simulink model "Microgrid"  (R2025b)
settings: Solver=FixedStepAuto  StartTime=0.0  StopTime=1  FixedStep=5e-7  RelTol=1e-3
InitFcn:
  | unitlmModelFile = get_param(bdroot, 'FileName');
  | if ~isempty(unitlmModelFile), addpath(fileparts(unitlmModelFile)); end
  | initialize_unitlm_microgrid();
  | clear unitlmModelFile
StopFcn:
  | %% StopFcn: save reference-system simulation results
  | 
  | % 获取模型文件所在目录
  | modelName = bdroot;
  | modelFile = get_param(modelName, 'FileName');
  | 
  | if isempty(modelFile)
  |     % 模型尚未保存时，使用当前工作目录
  |     modelDir = pwd;
  | else
  |     modelDir = fileparts(modelFile);
  | end
  | 
  | % 创建 result 文件夹
  | resultDir = fullfile(modelDir, 'result');
  | 
  | if ~exist(resultDir, 'dir')
  |     mkdir(resultDir);
  | end
  | 
  | % 需要保存的工作区变量
  | variableNames = {
  |     'server_voltage'
  |     'server_current'
  |     'server_PQ'
  |     'client_voltage'
  |     'client_current'
  |     'client_PQ'
  |     'client_omega'
  | };
  | 
  | % 用结构体保存，并添加 _ref 后缀
  | refData = struct();
  | 
  | for k = 1:numel(variableNames)
  | 
  |     originalName = variableNames{k};
  |     refName      = [originalName, '_ref'];
  | 
  |     % 检查变量是否存在于 Base Workspace
  |     variableExists = evalin( ...
  |         'base', ...
  |         sprintf('exist(''%s'', ''var'')', originalName));
  | 
  |     if variableExists
  |         refData.(refName) = evalin('base', originalName);
  |     else
  |         warning( ...
  |             'StopFcn:MissingVariable', ...
  |             'Variable "%s" was not found in the base workspace.', ...
  |             originalName);
  |     end
  | end
  | 
  | % 保存为 result/ref_system.mat
  | saveFile = fullfile(resultDir, 'ref_system.mat');
  | save(saveFile, '-struct', 'refData');
  | 
  | fprintf('Reference-system results saved to:\n%s\n', saveFile);
values from neighbouring files (symbols this model uses):
  Cf = Cf_pu*Cb    [initialize_unitlm_microgrid.m]
  f = logspace(log10(fMin), log10(fMax), nFrequency).'    [fit_non_heaviside_line_rational.m]    (also in initialize_unitlm_microgrid.m = 50)
  fsw1 = 10e3    (= 10000)    [initialize_unitlm_microgrid.m]
  gfm_AngleKi = 3    [initialize_unitlm_microgrid.m]
  gfm_AngleKp = 1.2    [initialize_unitlm_microgrid.m]
  gfm_PrefPu = 1.0    (= 1)    [initialize_unitlm_microgrid.m]
  gfm_VloopKi = 120    [initialize_unitlm_microgrid.m]
  gfm_VloopKp = 0.08    [initialize_unitlm_microgrid.m]
  gfm_VrefPu = 0.93    [initialize_unitlm_microgrid.m]
  Ip = 2*P/(3*Vp)    [initialize_unitlm_microgrid.m]
  L1 = L1_pu*Lb    [initialize_unitlm_microgrid.m]
  L2 = L2_pu*Lb    [initialize_unitlm_microgrid.m]
  L3 = L3_pu*Lb    [initialize_unitlm_microgrid.m]
  L4 = L4_pu*Lb    [initialize_unitlm_microgrid.m]
  Lc = Lc_pu*Lb    [initialize_unitlm_microgrid.m]
  Lf2 = Lf2_pu*Lb    [initialize_unitlm_microgrid.m]
  P = 5e6    (= 5000000)    [initialize_unitlm_microgrid.m]
  R1 = R1_pu*Zb    [initialize_unitlm_microgrid.m]
  R2 = R2_pu*Zb    [initialize_unitlm_microgrid.m]
  R3 = R3_pu*Zb    [initialize_unitlm_microgrid.m]
  R4 = R4_pu*Zb    [initialize_unitlm_microgrid.m]
  Rdamp = Rf    [initialize_unitlm_microgrid.m]
  Rf = Rf_pu*Zb    [initialize_unitlm_microgrid.m]
  Rload1 = Vp/Ip    [initialize_unitlm_microgrid.m]
  Rload2 = Vp/Ip    [initialize_unitlm_microgrid.m]
  Rload3 = Vp/Ip    [initialize_unitlm_microgrid.m]
  Rv_pu = 0.1    [initialize_unitlm_microgrid.m]
  Sxfmr = 6.3e6    (= 6300000)    [initialize_unitlm_microgrid.m]
  Vac = sqrt(2)*Vline/sqrt(3)    [initialize_unitlm_microgrid.m]
  Vdc = 1350    [initialize_unitlm_microgrid.m]
  Vhv = 66e3    (= 66000)    [initialize_unitlm_microgrid.m]
  Vline = 690    [initialize_unitlm_microgrid.m]
  Vp = Vac    [initialize_unitlm_microgrid.m]
  Wb = 2*pi*f    (= 314.159265359)    [initialize_unitlm_microgrid.m]
  Xv_pu = 0.3    [initialize_unitlm_microgrid.m]
undefined symbols (not defined in the file or in its folder): DiscIntNeverNeededParam, DPL, Lline1
libraries: spsThreePhaseSeriesRLCBranchLib x17, spsControlledVoltageSourceLib x9, spsabctodq0Lib x9, spsThreePhaseVIMeasurementLib x8, slpidlib x7, spsPower3phInstantaneousLib x4, spsThreePhaseBreakerLib x4, spsThreePhaseTransformerTwoWindingsLib x4, spsdq0toabcLib x3, SimplusGT x3, spsDCVoltageSourceLib x1, spsDistributedParametersLineLib x1
(part 3 of 3)

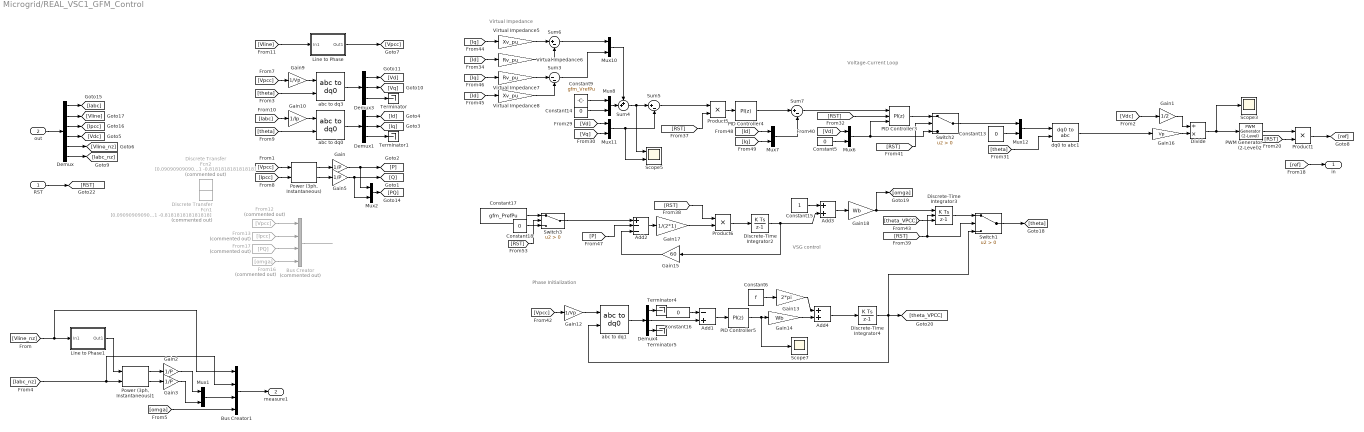
== system Microgrid/REAL_VSC1_GFM_Control ==
  note: Voltage-Current Loop
  note: VSG control
  note: Virtual Impedance
  note: Phase Initialization
  RST : Inport
  out : Inport  Port=2
  Add1 : Sum  Inputs=-+
  Add2 : Sum  Inputs=+--
  Add3 : Sum
  Add4 : Sum
  Bus Creator : BusCreator  Commented=on  Inputs=4
  Bus Creator1 : BusCreator  Inputs=4
  Constant{5,13..14,16} (4 alike) : Constant  Value=0
  Constant15 : Constant
  Constant17 : Constant  Value=gfm_PrefPu  SampleTime=-1
  Constant18 : Constant  Value=0  SampleTime=-1
  Constant6 : Constant  Value=f
  Constant9 : Constant  Value=gfm_VrefPu  SampleTime=-1
  Demux : Demux  Outputs=6
  Demux1 : Demux  Outputs=3
  Demux3 : Demux  Outputs=3
  Demux4 : Demux  Outputs=3
  Discrete Transfer Fcn1 : DiscreteTransferFcn  Commented=on  Numerator=[0.090909090909091 0.090909090909091]  Denominator=[1 -0.818181818181818]
  Discrete Transfer Fcn2 : DiscreteTransferFcn  Commented=on  Numerator=[0.090909090909091 0.090909090909091]  Denominator=[1 -0.818181818181818]
  Discrete-Time Integrator2 : DiscreteIntegrator  SampleTime=1/fsw1  ICPrevOutput=DiscIntNeverNeededParam  ICPrevScaledInput=DiscIntNeverNeededParam
  Discrete-Time Integrator3 : DiscreteIntegrator  ExternalReset=rising  InitialConditionSource=external  SampleTime=1/fsw1  ICPrevOutput=DiscIntNeverNeededParam  ICPrevScaledInput=DiscIntNeverNeededParam
  Discrete-Time Integrator4 : DiscreteIntegrator  SampleTime=1/fsw1  ICPrevOutput=DiscIntNeverNeededParam  ICPrevScaledInput=DiscIntNeverNeededParam
  Divide : Product  Inputs=/*
  From12 : From  Commented=on  GotoTag=Vpcc
  From13 : From  Commented=on  GotoTag=Ipcc
  From16 : From  Commented=on  GotoTag=omga
  From17 : From  Commented=on  GotoTag=PQ
  Gain{,2..3,5} (4 alike) : Gain  Gain=1/P
  Gain1 : Gain  Gain=1/2
  Gain10 : Gain  Gain=1/Ip
  Gain12 : Gain  Gain=1/Vp
  Gain13 : Gain  Gain=2*pi
  Gain14 : Gain  Gain=Wb
  Gain15 : Gain  Gain=60
  Gain16 : Gain  Gain=Vp
  Gain17 : Gain  Gain=1/(2*1)
  Gain18 : Gain  Gain=Wb
  Gain9 : Gain  Gain=1/Vp
  Line to Phase : Subsystem
  Line to Phase1 : Subsystem
  Mux{1..2,6..8,10..12} (8 alike) : Mux  Inputs=2
  PID Controller3 : slpidlib/PID Controller  Controller=PI  Form=Parallel  TimeDomain=Discrete-time  UseExternalTs=off  SampleTime=1/fsw1  IntegratorMethod=Forward Euler  FilterMethod=Forward Euler  ControllerParametersSource=internal  P=0.5  I=100  UseKiTs=off  D=0  UseExternalDerivativeSource=off  N=100  UseFilter=on  TunerSelectOption=Transfer Function Based (PID Tuner App)  InitialConditionSource=external  InitialConditionForIntegrator=0  InitialConditionForFilter=0  DifferentiatorICPrevScaledInput=0  ExternalReset=rising  TrackingMode=off  Kt=1  LimitOutput=off  SatLimitsSource=internal  UpperSaturationLimit=inf  LowerSaturationLimit=-inf  LinearizeAsGain=on  AntiWindupMode=none  Kb=1  LimitIntegrator=off  UpperIntegratorSaturationLimit=inf  LowerIntegratorSaturationLimit=-inf  POutMin=[]  POutMax=[]  IOutMin=[]  IOutMax=[]  DOutMin=[]  DOutMax=[]  NOutMin=[]  NOutMax=[]  SumOutMin=[]  SumOutMax=[]  SaturationOutMin=[]  SaturationOutMax=[]  PParamMin=[]  PParamMax=[]  IParamMin=[]  IParamMax=[]  DParamMin=[]  DParamMax=[]  NParamMin=[]  NParamMax=[]  KbParamMin=[]  KbParamMax=[]  KtParamMin=[]  KtParamMax=[]  KbOutMin=[]  KbOutMax=[]  KtOutMin=[]  KtOutMax=[]  IntegratorOutMin=[]  IntegratorOutMax=[]  FilterOutMin=[]  FilterOutMax=[]  SumI1OutMin=[]  SumI1OutMax=[]  SumI2OutMin=[]  SumI2OutMax=[]  SumI3OutMin=[]  SumI3OutMax=[]  SumI4OutMin=[]  SumI4OutMax=[]  SumDOutMin=[]  SumDOutMax=[]  DifferentiatorOutMin=[]  DifferentiatorOutMax=[]  FilterDiffOutCoefMin=[]  FilterDiffOutCoefMax=[]  ReciprocalOutMin=[]  ReciprocalOutMax=[]  SumDenOutMin=[]  SumDenOutMax=[]  SumNumOutMin=[]  SumNumOutMax=[]  DivideOutMin=[]  DivideOutMax=[]  UdiffTsProdOutMin=[]  UdiffTsProdOutMax=[]  NTsProdOutMin=[]  NTsProdOutMax=[]  UintegralTsProdOutMin=[]  UintegralTsProdOutMax=[]  UngainTsProdOutMin=[]  UngainTsProdOutMax=[]  ClampingZeroOutDataTypeStr=Inherit: Inherit via back propagation  ClampingZeroOutMin=[]  ClampingZeroOutMax=[]  FilterDenConstantOutDataTypeStr=Inherit: Inherit via back propagation  FilterDenConstantOutMin=[]  FilterDenConstantOutMax=[]  PCopyOutDataTypeStr=Inherit: Inherit via back propagation  PCopyOutMin=[]  PCopyOutMax=[]  NCopyOutDataTypeStr=Inherit: Inherit via back propagation  NCopyOutMin=[]  NCopyOutMax=[]  IntegratorContinuousStateAttributes=''  IntegratorStateMustResolveToSignalObject=off  IntegratorRTWStateStorageClass=Auto  FilterContinuousStateAttributes=''  FilterStateMustResolveToSignalObject=off  FilterRTWStateStorageClass=Auto  ParallelPVariant=InternalParameters  IdealPVariant=Disabled  IVariant=InternalParameters  DVariant=Disabled  IntegratorVariant=Discrete  SatVariant=Disabled  AWVariant=Passthrough  PCopyVariant=Disabled  TRVariant=Disabled  FdbkBlocksVariant=Forward  IdealPFdbkVariant=Disabled  SatFdbkVariant=Disabled  DerivativeFilterVariant=Disabled  NVariant=Disabled  NCopyVariant=Disabled_SignalSpec  FilterICVariant=Disabled  IntegratorICVariant=ExternalICs  ExternalResetVariant=ExternalReset  TRSumVariant=Passthrough  SumFdbkVariant=Disabled  SumVariant=Sum_PI  TsampFilterVariant=InternalTs  TsampNgainVariant=Passthrough  TsampIntegralVariant=Disabled_SignalSpec  ExternalSaturationOutDataTypeStr=Inherit: Same as second input  DerivativeSourceVariant=Disabled  PreIntVariant=InternalPreInt
  PID Controller4 : slpidlib/PID Controller  Controller=PI  Form=Parallel  TimeDomain=Discrete-time  UseExternalTs=off  SampleTime=1/fsw1  IntegratorMethod=Forward Euler  FilterMethod=Forward Euler  ControllerParametersSource=internal  P=gfm_VloopKp  I=gfm_VloopKi  UseKiTs=off  D=0  UseExternalDerivativeSource=off  N=100  UseFilter=on  TunerSelectOption=Transfer Function Based (PID Tuner App)  InitialConditionSource=internal  InitialConditionForIntegrator=0  InitialConditionForFilter=0  DifferentiatorICPrevScaledInput=0  ExternalReset=none  TrackingMode=off  Kt=1  LimitOutput=off  SatLimitsSource=internal  UpperSaturationLimit=inf  LowerSaturationLimit=-inf  LinearizeAsGain=on  AntiWindupMode=none  Kb=1  LimitIntegrator=off  UpperIntegratorSaturationLimit=inf  LowerIntegratorSaturationLimit=-inf  POutMin=[]  POutMax=[]  IOutMin=[]  IOutMax=[]  DOutMin=[]  DOutMax=[]  NOutMin=[]  NOutMax=[]  SumOutMin=[]  SumOutMax=[]  SaturationOutMin=[]  SaturationOutMax=[]  PParamMin=[]  PParamMax=[]  IParamMin=[]  IParamMax=[]  DParamMin=[]  DParamMax=[]  NParamMin=[]  NParamMax=[]  KbParamMin=[]  KbParamMax=[]  KtParamMin=[]  KtParamMax=[]  KbOutMin=[]  KbOutMax=[]  KtOutMin=[]  KtOutMax=[]  IntegratorOutMin=[]  IntegratorOutMax=[]  FilterOutMin=[]  FilterOutMax=[]  SumI1OutMin=[]  SumI1OutMax=[]  SumI2OutMin=[]  SumI2OutMax=[]  SumI3OutMin=[]  SumI3OutMax=[]  SumI4OutMin=[]  SumI4OutMax=[]  SumDOutMin=[]  SumDOutMax=[]  DifferentiatorOutMin=[]  DifferentiatorOutMax=[]  FilterDiffOutCoefMin=[]  FilterDiffOutCoefMax=[]  ReciprocalOutMin=[]  ReciprocalOutMax=[]  SumDenOutMin=[]  SumDenOutMax=[]  SumNumOutMin=[]  SumNumOutMax=[]  DivideOutMin=[]  DivideOutMax=[]  UdiffTsProdOutMin=[]  UdiffTsProdOutMax=[]  NTsProdOutMin=[]  NTsProdOutMax=[]  UintegralTsProdOutMin=[]  UintegralTsProdOutMax=[]  UngainTsProdOutMin=[]  UngainTsProdOutMax=[]  ClampingZeroOutDataTypeStr=Inherit: Inherit via back propagation  ClampingZeroOutMin=[]  ClampingZeroOutMax=[]  FilterDenConstantOutDataTypeStr=Inherit: Inherit via back propagation  FilterDenConstantOutMin=[]  FilterDenConstantOutMax=[]  PCopyOutDataTypeStr=Inherit: Inherit via back propagation  PCopyOutMin=[]  PCopyOutMax=[]  NCopyOutDataTypeStr=Inherit: Inherit via back propagation  NCopyOutMin=[]  NCopyOutMax=[]  IntegratorContinuousStateAttributes=''  IntegratorStateMustResolveToSignalObject=off  IntegratorRTWStateStorageClass=Auto  FilterContinuousStateAttributes=''  FilterStateMustResolveToSignalObject=off  FilterRTWStateStorageClass=Auto  ParallelPVariant=InternalParameters  IdealPVariant=Disabled  IVariant=InternalParameters  DVariant=Disabled  IntegratorVariant=Discrete  SatVariant=Disabled  AWVariant=Passthrough  PCopyVariant=Disabled  TRVariant=Disabled  FdbkBlocksVariant=Forward  IdealPFdbkVariant=Disabled  SatFdbkVariant=Disabled  DerivativeFilterVariant=Disabled  NVariant=Disabled  NCopyVariant=Disabled_SignalSpec  FilterICVariant=Disabled  IntegratorICVariant=InternalICs  ExternalResetVariant=Disabled  TRSumVariant=Passthrough  SumFdbkVariant=Disabled  SumVariant=Sum_PI  TsampFilterVariant=InternalTs  TsampNgainVariant=Passthrough  TsampIntegralVariant=Disabled_SignalSpec  ExternalSaturationOutDataTypeStr=Inherit: Same as second input  DerivativeSourceVariant=Disabled  PreIntVariant=InternalPreInt
  PID Controller5 : slpidlib/PID Controller  Controller=PI  Form=Parallel  TimeDomain=Discrete-time  UseExternalTs=off  SampleTime=1/fsw1  IntegratorMethod=Forward Euler  FilterMethod=Forward Euler  ControllerParametersSource=internal  P=gfm_AngleKp  I=gfm_AngleKi  UseKiTs=off  D=0  UseExternalDerivativeSource=off  N=100  UseFilter=on  TunerSelectOption=Transfer Function Based (PID Tuner App)  InitialConditionSource=internal  InitialConditionForIntegrator=0  InitialConditionForFilter=0  DifferentiatorICPrevScaledInput=0  ExternalReset=none  TrackingMode=off  Kt=1  LimitOutput=off  SatLimitsSource=internal  UpperSaturationLimit=inf  LowerSaturationLimit=-inf  LinearizeAsGain=on  AntiWindupMode=none  Kb=1  LimitIntegrator=off  UpperIntegratorSaturationLimit=inf  LowerIntegratorSaturationLimit=-inf  POutMin=[]  POutMax=[]  IOutMin=[]  IOutMax=[]  DOutMin=[]  DOutMax=[]  NOutMin=[]  NOutMax=[]  SumOutMin=[]  SumOutMax=[]  SaturationOutMin=[]  SaturationOutMax=[]  PParamMin=[]  PParamMax=[]  IParamMin=[]  IParamMax=[]  DParamMin=[]  DParamMax=[]  NParamMin=[]  NParamMax=[]  KbParamMin=[]  KbParamMax=[]  KtParamMin=[]  KtParamMax=[]  KbOutMin=[]  KbOutMax=[]  KtOutMin=[]  KtOutMax=[]  IntegratorOutMin=[]  IntegratorOutMax=[]  FilterOutMin=[]  FilterOutMax=[]  SumI1OutMin=[]  SumI1OutMax=[]  SumI2OutMin=[]  SumI2OutMax=[]  SumI3OutMin=[]  SumI3OutMax=[]  SumI4OutMin=[]  SumI4OutMax=[]  SumDOutMin=[]  SumDOutMax=[]  DifferentiatorOutMin=[]  DifferentiatorOutMax=[]  FilterDiffOutCoefMin=[]  FilterDiffOutCoefMax=[]  ReciprocalOutMin=[]  ReciprocalOutMax=[]  SumDenOutMin=[]  SumDenOutMax=[]  SumNumOutMin=[]  SumNumOutMax=[]  DivideOutMin=[]  DivideOutMax=[]  UdiffTsProdOutMin=[]  UdiffTsProdOutMax=[]  NTsProdOutMin=[]  NTsProdOutMax=[]  UintegralTsProdOutMin=[]  UintegralTsProdOutMax=[]  UngainTsProdOutMin=[]  UngainTsProdOutMax=[]  ClampingZeroOutDataTypeStr=Inherit: Inherit via back propagation  ClampingZeroOutMin=[]  ClampingZeroOutMax=[]  FilterDenConstantOutDataTypeStr=Inherit: Inherit via back propagation  FilterDenConstantOutMin=[]  FilterDenConstantOutMax=[]  PCopyOutDataTypeStr=Inherit: Inherit via back propagation  PCopyOutMin=[]  PCopyOutMax=[]  NCopyOutDataTypeStr=Inherit: Inherit via back propagation  NCopyOutMin=[]  NCopyOutMax=[]  IntegratorContinuousStateAttributes=''  IntegratorStateMustResolveToSignalObject=off  IntegratorRTWStateStorageClass=Auto  FilterContinuousStateAttributes=''  FilterStateMustResolveToSignalObject=off  FilterRTWStateStorageClass=Auto  ParallelPVariant=InternalParameters  IdealPVariant=Disabled  IVariant=InternalParameters  DVariant=Disabled  IntegratorVariant=Discrete  SatVariant=Disabled  AWVariant=Passthrough  PCopyVariant=Disabled  TRVariant=Disabled  FdbkBlocksVariant=Forward  IdealPFdbkVariant=Disabled  SatFdbkVariant=Disabled  DerivativeFilterVariant=Disabled  NVariant=Disabled  NCopyVariant=Disabled_SignalSpec  FilterICVariant=Disabled  IntegratorICVariant=InternalICs  ExternalResetVariant=Disabled  TRSumVariant=Passthrough  SumFdbkVariant=Disabled  SumVariant=Sum_PI  TsampFilterVariant=InternalTs  TsampNgainVariant=Passthrough  TsampIntegralVariant=Disabled_SignalSpec  ExternalSaturationOutDataTypeStr=Inherit: Same as second input  DerivativeSourceVariant=Disabled  PreIntVariant=InternalPreInt
  PWM Generator (2-Level)2 : spsPWMGenerator2LevelLib/PWM Generator (2-Level)  ModulatorType=Three-phase bridge (6 pulses)  ModulatorMode=Unsynchronized  Fc=fsw1  Pc=0  nF=27  MinMax="[ -1  1 ]"  SamplingTechnique=Asymmetrical regular (double edge)  ModulatingSignals=off  m=0.8  Freq=60  Phase=0  Ts=0  ShowCarrierOutport=off
  "Power (3ph, Instantaneous)" : spsPower3phInstantaneousLib/Power (3ph, Instantaneous)
  "Power (3ph, Instantaneous)1" : spsPower3phInstantaneousLib/Power (3ph, Instantaneous)
  Product1 : Product
  Product5 : Product
  Product6 : Product
  Scope3 : Scope
      settings: ActiveDisplayYMinimum=-0.017929362342912838  ActiveDisplayYMaximum=0.017670248495709841
  Scope5 : Scope  NumInputPorts=2
      settings: ActiveDisplayYMinimum=-0.89875  ActiveDisplayYMaximum=1.61871
  Scope7 : Scope
      settings: ActiveDisplayYMinimum=-0.17841  ActiveDisplayYMaximum=0.07598  DataLoggingVariableName=ScopeData3
  Sum3 : Sum  Inputs=|--
  Sum4 : Sum  Inputs=++|
  Sum5 : Sum  Inputs=|+-
  Sum6 : Sum  Inputs=|+-
  Sum7 : Sum  Inputs=|+-
  Switch1 : Switch  Criteria=u2 > Threshold  SaturateOnIntegerOverflow=off  InputSameDT=off
  Switch2 : Switch  Criteria=u2 > Threshold  SaturateOnIntegerOverflow=off  InputSameDT=off
  Switch3 : Switch  Criteria=u2 > Threshold  SaturateOnIntegerOverflow=off  InputSameDT=off
  Terminator{,1,4..5} (4 alike) : Terminator
  Virtual Impedance5 : Gain  Gain=Xv_pu
  Virtual Impedance6 : Gain  Gain=Rv_pu
  Virtual Impedance7 : Gain  Gain=Rv_pu
  Virtual Impedance8 : Gain  Gain=Xv_pu
  abc to dq0 : spsabctodq0Lib/abc to dq0  Alignment=90 degrees behind phase A axis
  abc to dq1 : spsabctodq0Lib/abc to dq0  Alignment=90 degrees behind phase A axis
  abc to dq3 : spsabctodq0Lib/abc to dq0  Alignment=90 degrees behind phase A axis
  dq0 to abc1 : spsdq0toabcLib/dq0 to abc  Alignment=90 degrees behind phase A axis
  in : Outport
  measure1 : Outport  Port=2
  wires:
  [RST] -> Product1/2
  Gain16/1 -> Divide/2
  PWM Generator (2-Level)2/1 -> Product1/1
  Product1/1 -> [ref]
  Gain1/1 -> Divide/1
  Divide/1 -> PWM Generator (2-Level)2/1, Scope3/1
  [Vdc] -> Gain1/1
  [ref] -> in/1
  Gain5/1 -> [Q], Mux2/2
  Gain/1 -> [P], Mux2/1
  Line to Phase/1(Out1) -> [Vpcc]
  [Vline] -> Line to Phase/1(In1)
  Demux1/2 -> [Iq]
  Demux1/3 -> Terminator1/1
  Demux1/1 -> [Id]
  abc to dq0/1 -> Demux1/1
  [Iabc] -> Gain10/1
  Gain9/1 -> abc to dq3/1
  abc to dq3/1 -> Demux3/1
  Gain10/1 -> abc to dq0/1
  Demux3/1 -> [Vd]
  [theta] -> abc to dq0/2
  [theta] -> abc to dq3/2
  Demux3/3 -> Terminator/1
  [Vpcc] -> Gain9/1
  Demux3/2 -> [Vq]
  [Vpcc] -> "Power (3ph, Instantaneous)"/1
  [Ipcc] -> "Power (3ph, Instantaneous)"/2
  "Power (3ph, Instantaneous)"/2 -> Gain5/1
  "Power (3ph, Instantaneous)"/1 -> Gain/1
  Mux2/1 -> [PQ]
  out/1 -> Demux/1
  Demux/3 -> [Ipcc]
  Demux/2 -> [Vline]
  Demux/1 -> [Iabc]
  Demux/4 -> [Vdc]
  Constant14/1 -> Mux8/2
  Constant13/1 -> Mux12/2
  Mux8/1 -> Sum4/2
  Discrete-Time Integrator2/1 -> Add3/2, Gain15/1
  [Iq] -> Mux7/2
  Add2/1 -> Gain17/1
  Gain15/1 -> Add2/3
  Switch3/1 -> Add2/1
  Add3/1 -> Gain18/1
  [Vq] -> Mux11/2
  [Id] -> Mux7/1
  [Vd] -> Mux11/1
  Sum5/1 -> Product5/1
  [P] -> Add2/2
  Mux10/1 -> Sum4/1
  Product5/1 -> PID Controller4/1
  dq0 to abc1/1 -> Gain16/1
  Constant6/1 -> Gain13/1
  Demux4/3 -> Terminator5/1
  Gain17/1 -> Product6/2
  [RST] -> PID Controller3/2
  abc to dq1/1 -> Demux4/1
  [RST] -> Switch1/2, Discrete-Time Integrator3/2
  Constant16/1 -> Add1/1
  [RST] -> Product5/2
  PID Controller4/1 -> Sum7/1
  Add1/1 -> PID Controller5/1
  Sum4/1 -> Scope5/1, Sum5/1
  [Id] -> Virtual Impedance6/1
  Virtual Impedance8/1 -> Sum3/2
  Mux7/1 -> Sum7/2
  Demux4/1 -> Terminator4/1
  Demux4/2 -> Add1/2
  Switch1/1 -> [theta]
  Discrete-Time Integrator4/1 -> Switch1/3, [theta_VPCC], abc to dq1/2
  Virtual Impedance7/1 -> Sum3/1
  Constant9/1 -> Mux8/1
  [RST] -> Switch2/2
  Add4/1 -> Discrete-Time Integrator4/1
  [Iq] -> Virtual Impedance5/1
  Sum6/1 -> Mux10/1
  [theta] -> dq0 to abc1/2
  [Iq] -> Virtual Impedance7/1
  Product6/1 -> Discrete-Time Integrator2/1
  Virtual Impedance6/1 -> Sum6/2
  Discrete-Time Integrator3/1 -> Switch1/1
  PID Controller3/1 -> Switch2/1
  Gain14/1 -> Add4/2
  [Vpcc] -> Gain12/1
  RST/1 -> [RST]
  Mux12/1 -> dq0 to abc1/1
  Mux6/1 -> Switch2/3, PID Controller3/3
  Virtual Impedance5/1 -> Sum6/1
  [RST] -> Product6/1
  Gain12/1 -> abc to dq1/1
  Sum3/1 -> Mux10/2
  Gain13/1 -> Add4/1
  [Vd] -> Mux6/1
  Mux11/1 -> Sum5/2, Scope5/2
  Gain18/1 -> Discrete-Time Integrator3/1, [omga]
  [Id] -> Virtual Impedance8/1
  Constant5/1 -> Mux6/2
  PID Controller5/1 -> Scope7/1, Gain14/1
  [theta_VPCC] -> Discrete-Time Integrator3/3
  Constant15/1 -> Add3/1
  Constant17/1 -> Switch3/1
  Constant18/1 -> Switch3/3
  [RST] -> Switch3/2
  Bus Creator/1 -> ?
  From12/1 -> Bus Creator/1
  From13/1 -> Bus Creator/2
  From17/1 -> Bus Creator/3
  From16/1 -> Bus Creator/4
  Sum7/1 -> PID Controller3/1
  Switch2/1 -> Mux12/1
  "Power (3ph, Instantaneous)1"/1 -> Gain2/1
  Mux1/1 -> Bus Creator1/3
  Gain2/1 -> Mux1/1
  "Power (3ph, Instantaneous)1"/2 -> Gain3/1
  Bus Creator1/1 -> measure1/1
  [omga] -> Bus Creator1/4
  Line to Phase1/1(Out1) -> "Power (3ph, Instantaneous)1"/1
  Gain3/1 -> Mux1/2
  [Iabc_nz] -> Bus Creator1/2, "Power (3ph, Instantaneous)1"/2
  [Vline_nz] -> Bus Creator1/1, Line to Phase1/1(In1)
  Demux/5 -> [Vline_nz]
  Demux/6 -> [Iabc_nz]

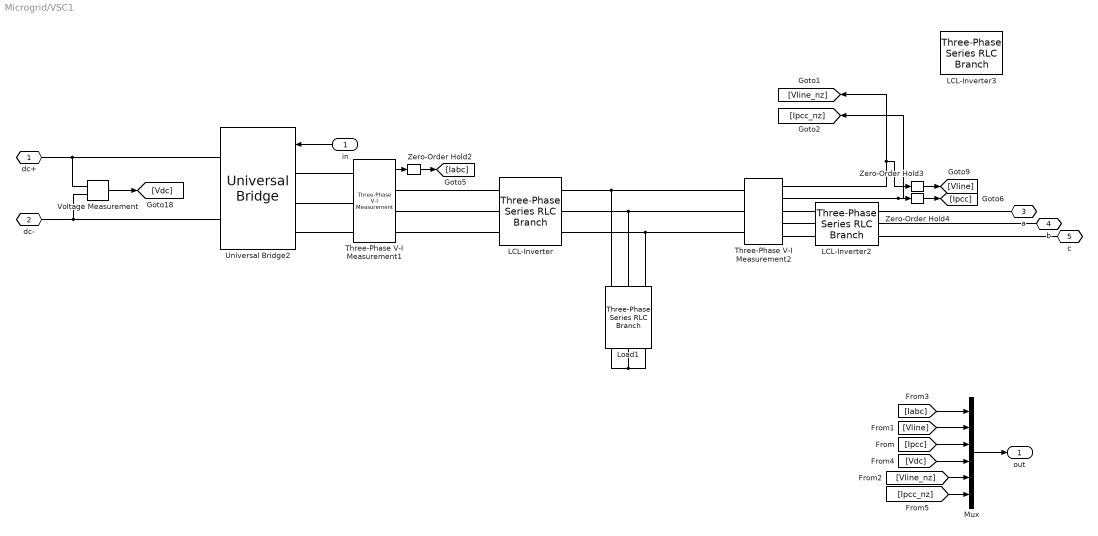
== system Microgrid/VSC1 ==
  in : Inport
  LCL-Inverter : spsThreePhaseSeriesRLCBranchLib/Three-Phase Series RLC Branch  LConnTagsString=A|B|C  RConnTagsString=A|B|C  BranchType=RL  Resistance=Rf  Inductance=Lc  Capacitance=1e-6  Measurements=None
  LCL-Inverter2 : spsThreePhaseSeriesRLCBranchLib/Three-Phase Series RLC Branch  LConnTagsString=A|B|C  RConnTagsString=A|B|C  BranchType=RL  Resistance=Rf  Inductance=Lf2  Capacitance=1e-6  Measurements=None
  LCL-Inverter3 : spsThreePhaseSeriesRLCBranchLib/Three-Phase Series RLC Branch  LConnTagsString=A|B|C  RConnTagsString=A|B|C  BranchType=RL  Resistance=Rf  Inductance=Lf2  Capacitance=1e-6  Measurements=None
  Load1 : spsThreePhaseSeriesRLCBranchLib/Three-Phase Series RLC Branch  LConnTagsString=A|B|C  RConnTagsString=A|B|C  BranchType=RC  Resistance=Rdamp  Inductance=1e-3  Capacitance=Cf  Measurements=None
  Mux : Mux  Inputs=6
  Three-Phase V-I Measurement1 : spsThreePhaseVIMeasurementLib/Three-Phase V-I Measurement  VoltageMeasurement=no  SetLabelV=off  LabelV=Vabc  Vpu=off  VpuLL=off  CurrentMeasurement=yes  SetLabelI=off  LabelI=Iabc  Ipu=off  Pbase=100e6  Vbase=500e3  OutputType=Complex  PhasorSimulation=off  PSBequivalent=0
  Three-Phase V-I Measurement2 : spsThreePhaseVIMeasurementLib/Three-Phase V-I Measurement  VoltageMeasurement=phase-to-phase  SetLabelV=off  LabelV=Vabc  Vpu=off  VpuLL=off  CurrentMeasurement=yes  SetLabelI=off  LabelI=Iabc  Ipu=off  Pbase=100e6  Vbase=500e3  OutputType=Complex  PhasorSimulation=off  PSBequivalent=0
  Universal Bridge2 : spsUniversalBridgeLib/Universal Bridge  Arms=3  SnubberResistance=1e5  SnubberCapacitance=inf  Device=IGBT / Diodes  Ron=RonVSC  Lon=0  ForwardVoltages="[  0  0  ]"  ForwardVoltage=0  GTOparameters=[ 10e-6 , 20e-6 ]  IGBTparameters=[ 1e-6 , 2e-6 ]  Measurements=None  Measurements_2=None  converterType=Rectifier
  Voltage Measurement : spsVoltageMeasurementLib/Voltage Measurement  PhasorSimulation=off  OutputType=Complex  PSBequivalent=0
  Zero-Order Hold2 : ZeroOrderHold  SampleTime=1/fsw1
  Zero-Order Hold3 : ZeroOrderHold  SampleTime=1/fsw1
  Zero-Order Hold4 : ZeroOrderHold  SampleTime=1/fsw1
  dc+ : PMIOPort  Side=Left
  dc- : PMIOPort  Port=2  Side=Left
  a : PMIOPort  Port=3  Side=Right
  b : PMIOPort  Port=4  Side=Right
  c : PMIOPort  Port=5  Side=Right
  out : Outport
  wires:
  Zero-Order Hold4/1 -> [Ipcc]
  Zero-Order Hold3/1 -> [Vline]
  Three-Phase V-I Measurement1/1 -> Zero-Order Hold2/1
  in/1 -> Universal Bridge2/1
  Zero-Order Hold2/1 -> [Iabc]
  [Vdc] -> Mux/4
  [Ipcc] -> Mux/3
  [Vline] -> Mux/2
  [Iabc] -> Mux/1
  Mux/1 -> out/1
  Voltage Measurement/1 -> [Vdc]
  [Vline_nz] -> Mux/5
  [Ipcc_nz] -> Mux/6
  Three-Phase V-I Measurement2/1 -> Zero-Order Hold3/1, [Vline_nz]
  Three-Phase V-I Measurement2/2 -> [Ipcc_nz], Zero-Order Hold4/1
  connections:
  Load1/RConn2 -- Load1/RConn1 -- Load1/RConn3
  Load1/LConn2 -- Three-Phase V-I Measurement2/LConn2 -- LCL-Inverter/RConn2
  Load1/LConn1 -- Three-Phase V-I Measurement2/LConn1 -- LCL-Inverter/RConn1
  Load1/LConn3 -- Three-Phase V-I Measurement2/LConn3 -- LCL-Inverter/RConn3
  Universal Bridge2/LConn3 -- Three-Phase V-I Measurement1/LConn3
  Three-Phase V-I Measurement1/RConn1 -- LCL-Inverter/LConn1
  Three-Phase V-I Measurement1/RConn2 -- LCL-Inverter/LConn2
  Universal Bridge2/LConn1 -- Three-Phase V-I Measurement1/LConn1
  Universal Bridge2/LConn2 -- Three-Phase V-I Measurement1/LConn2
  Three-Phase V-I Measurement1/RConn3 -- LCL-Inverter/LConn3
  Universal Bridge2/RConn1 -- Voltage Measurement/LConn1 -- dc+/RConn1
  Universal Bridge2/RConn2 -- Voltage Measurement/LConn2 -- dc-/RConn1
  LCL-Inverter2/LConn1 -- Three-Phase V-I Measurement2/RConn1
  LCL-Inverter2/LConn2 -- Three-Phase V-I Measurement2/RConn2
  LCL-Inverter2/LConn3 -- Three-Phase V-I Measurement2/RConn3
  LCL-Inverter2/RConn1 -- a/RConn1
  LCL-Inverter2/RConn2 -- b/RConn1
  LCL-Inverter2/RConn3 -- c/RConn1

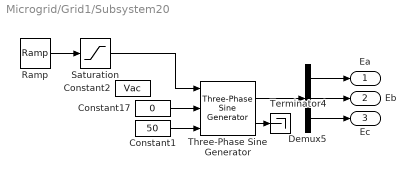
== system Microgrid/Grid1/Subsystem20 ==
  Constant1 : Constant  Value=50
  Constant17 : Constant  Value=0
  Constant2 : Constant  Value=Vac
  Demux5 : Demux  Outputs=3
  Ramp : simulink/Sources/Ramp  slope=Vac/0.01  start=0  InitialOutput=0
  Saturation : Saturate  UpperLimit=Vac  LowerLimit=0
  Terminator4 : Terminator
  Three-Phase Sine Generator : spsThreePhaseSineGeneratorLib/Three-Phase Sine Generator  Ts=1e-6
      settings: LibrarySourceBlock=|
      | sps_lib/Sources/Signal Generator Sources/Three-Phase
      | Sine Generator
  Ea : Outport
  Eb : Outport  Port=2
  Ec : Outport  Port=3
  wires:
  Three-Phase Sine Generator/1 -> Demux5/1
  Three-Phase Sine Generator/2 -> Terminator4/1
  Demux5/1 -> Ea/1
  Demux5/2 -> Eb/1
  Demux5/3 -> Ec/1
  Constant17/1 -> Three-Phase Sine Generator/2
  Constant1/1 -> Three-Phase Sine Generator/3
  Ramp/1 -> Saturation/1
  Saturation/1 -> Three-Phase Sine Generator/1

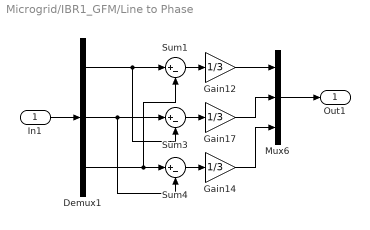
== system Microgrid/IBR1_GFM/Line to Phase ==
  In1 : Inport
  Demux1 : Demux  Outputs=3
  Gain12 : Gain  Gain=1/3
  Gain14 : Gain  Gain=1/3
  Gain17 : Gain  Gain=1/3
  Mux6 : Mux  Inputs=3
  Sum1 : Sum  Inputs=|+-
  Sum3 : Sum  Inputs=|+-
  Sum4 : Sum  Inputs=|+-
  Out1 : Outport
  wires:
  Sum3/1 -> Gain17/1
  Gain17/1 -> Mux6/2
  In1/1 -> Demux1/1
  Gain14/1 -> Mux6/3
  Sum1/1 -> Gain12/1
  Sum4/1 -> Gain14/1
  Demux1/3 -> Sum4/1, Sum1/2
  Demux1/2 -> Sum4/2, Sum3/1
  Gain12/1 -> Mux6/1
  Mux6/1 -> Out1/1
  Demux1/1 -> Sum3/2, Sum1/1

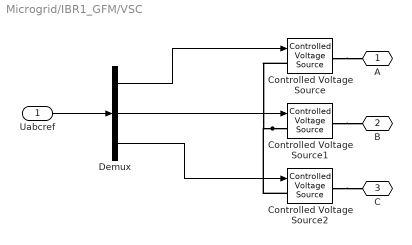
== system Microgrid/IBR1_GFM/VSC ==
  Uabcref : Inport
  Controlled Voltage Source : spsControlledVoltageSourceLib/Controlled Voltage Source  Initialize=on  Source_Type=AC  Amplitude=0  Phase=0  Frequency=0  Measurements=None
  Controlled Voltage Source1 : spsControlledVoltageSourceLib/Controlled Voltage Source  Initialize=on  Source_Type=AC  Amplitude=0  Phase=0  Frequency=0  Measurements=None
  Controlled Voltage Source2 : spsControlledVoltageSourceLib/Controlled Voltage Source  Initialize=on  Source_Type=AC  Amplitude=0  Phase=0  Frequency=0  Measurements=None
  Demux : Demux  Outputs=3
  A : PMIOPort  Side=Right
  B : PMIOPort  Port=2  Side=Right
  C : PMIOPort  Port=3  Side=Right
  wires:
  Demux/2 -> Controlled Voltage Source1/1
  Uabcref/1 -> Demux/1
  Demux/1 -> Controlled Voltage Source/1
  Demux/3 -> Controlled Voltage Source2/1
  connections:
  Controlled Voltage Source2/RConn1 -- C/RConn1
  Controlled Voltage Source1/LConn1 -- Controlled Voltage Source2/LConn1 -- Controlled Voltage Source/LConn1
  Controlled Voltage Source1/RConn1 -- B/RConn1
  Controlled Voltage Source/RConn1 -- A/RConn1

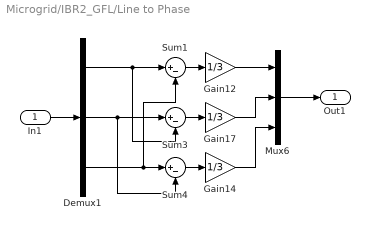
== system Microgrid/IBR2_GFL/Line to Phase ==
  In1 : Inport
  Demux1 : Demux  Outputs=3
  Gain12 : Gain  Gain=1/3
  Gain14 : Gain  Gain=1/3
  Gain17 : Gain  Gain=1/3
  Mux6 : Mux  Inputs=3
  Sum1 : Sum  Inputs=|+-
  Sum3 : Sum  Inputs=|+-
  Sum4 : Sum  Inputs=|+-
  Out1 : Outport
  wires:
  Sum3/1 -> Gain17/1
  Gain17/1 -> Mux6/2
  In1/1 -> Demux1/1
  Gain14/1 -> Mux6/3
  Sum1/1 -> Gain12/1
  Sum4/1 -> Gain14/1
  Demux1/3 -> Sum4/1, Sum1/2
  Demux1/2 -> Sum4/2, Sum3/1
  Gain12/1 -> Mux6/1
  Mux6/1 -> Out1/1
  Demux1/1 -> Sum3/2, Sum1/1

== system Microgrid/IBR2_GFL/PID ==
  In1 : Inport
  Discrete-Time Integrator : DiscreteIntegrator  gainval=5  SampleTime=-1  LimitOutput=on  UpperSaturationLimit=1.5  LowerSaturationLimit=-1.5  ICPrevOutput=DiscIntNeverNeededParam  ICPrevScaledInput=DiscIntNeverNeededParam
  Gain2 : Gain  SaturateOnIntegerOverflow=on  OutDataTypeStr=Inherit: Same as input  ParamDataTypeStr=Inherit: Same as input
  Saturation : Saturate  UpperLimit=1.5  LowerLimit=-1.5
  Sum2 : Sum  Inputs=++|
  Out1 : Outport  VectorParamsAs1DForOutWhenUnconnected=off
  wires:
  Gain2/1 -> Sum2/2
  In1/1 -> Discrete-Time Integrator/1, Gain2/1
  Sum2/1 -> Saturation/1
  Discrete-Time Integrator/1 -> Sum2/1
  Saturation/1 -> Out1/1

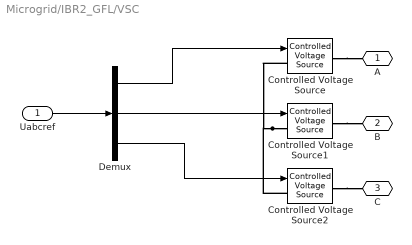
== system Microgrid/IBR2_GFL/VSC ==
  Uabcref : Inport
  Controlled Voltage Source : spsControlledVoltageSourceLib/Controlled Voltage Source  Initialize=on  Source_Type=AC  Amplitude=0  Phase=0  Frequency=0  Measurements=None
  Controlled Voltage Source1 : spsControlledVoltageSourceLib/Controlled Voltage Source  Initialize=on  Source_Type=AC  Amplitude=0  Phase=0  Frequency=0  Measurements=None
  Controlled Voltage Source2 : spsControlledVoltageSourceLib/Controlled Voltage Source  Initialize=on  Source_Type=AC  Amplitude=0  Phase=0  Frequency=0  Measurements=None
  Demux : Demux  Outputs=3
  A : PMIOPort  Side=Right
  B : PMIOPort  Port=2  Side=Right
  C : PMIOPort  Port=3  Side=Right
  wires:
  Demux/2 -> Controlled Voltage Source1/1
  Uabcref/1 -> Demux/1
  Demux/1 -> Controlled Voltage Source/1
  Demux/3 -> Controlled Voltage Source2/1
  connections:
  Controlled Voltage Source2/RConn1 -- C/RConn1
  Controlled Voltage Source1/LConn1 -- Controlled Voltage Source/LConn1 -- Controlled Voltage Source2/LConn1
  Controlled Voltage Source1/RConn1 -- B/RConn1
  Controlled Voltage Source/RConn1 -- A/RConn1

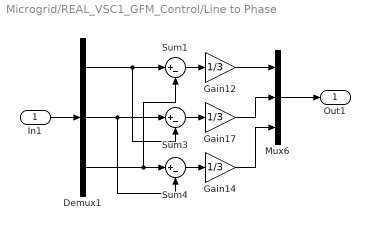
== system Microgrid/REAL_VSC1_GFM_Control/Line to Phase ==
  In1 : Inport
  Demux1 : Demux  Outputs=3
  Gain12 : Gain  Gain=1/3
  Gain14 : Gain  Gain=1/3
  Gain17 : Gain  Gain=1/3
  Mux6 : Mux  Inputs=3
  Sum1 : Sum  Inputs=|+-
  Sum3 : Sum  Inputs=|+-
  Sum4 : Sum  Inputs=|+-
  Out1 : Outport
  wires:
  Demux1/1 -> Sum1/1, Sum3/2
  Mux6/1 -> Out1/1
  Gain12/1 -> Mux6/1
  Demux1/2 -> Sum3/1, Sum4/2
  Demux1/3 -> Sum1/2, Sum4/1
  Sum4/1 -> Gain14/1
  Sum1/1 -> Gain12/1
  Gain14/1 -> Mux6/3
  In1/1 -> Demux1/1
  Gain17/1 -> Mux6/2
  Sum3/1 -> Gain17/1

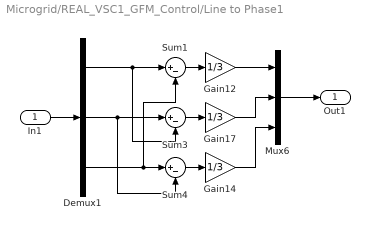
== system Microgrid/REAL_VSC1_GFM_Control/Line to Phase1 ==
  In1 : Inport
  Demux1 : Demux  Outputs=3
  Gain12 : Gain  Gain=1/3
  Gain14 : Gain  Gain=1/3
  Gain17 : Gain  Gain=1/3
  Mux6 : Mux  Inputs=3
  Sum1 : Sum  Inputs=|+-
  Sum3 : Sum  Inputs=|+-
  Sum4 : Sum  Inputs=|+-
  Out1 : Outport
  wires:
  Sum3/1 -> Gain17/1
  Gain17/1 -> Mux6/2
  In1/1 -> Demux1/1
  Gain14/1 -> Mux6/3
  Sum1/1 -> Gain12/1
  Sum4/1 -> Gain14/1
  Demux1/3 -> Sum4/1, Sum1/2
  Demux1/2 -> Sum4/2, Sum3/1
  Gain12/1 -> Mux6/1
  Mux6/1 -> Out1/1
  Demux1/1 -> Sum3/2, Sum1/1
